simulink model "seventh"  (R2020a)
settings: Solver=VariableStepAuto  StartTime=0.0  StopTime=10.0  RelTol=1e-3
model workspace (MAT data in the model file):
  A = Simulink.Parameter
  A.Value = 1
  A.DataType = 'auto'
  A.Dimensions = [1 1]
  B = Simulink.Parameter
  B.Value = 2
  B.DataType = 'auto'
  B.Dimensions = [1 1]
  C = Simulink.Parameter
  C.Value = -1
  C.DataType = 'auto'
  C.Dimensions = [1 1]
  D = Simulink.Parameter
  D.Value = 1
  D.DataType = 'auto'
  D.Dimensions = [1 1]
  E = Simulink.Parameter
  E.Value = 1
  E.DataType = 'auto'
  E.Dimensions = [1 1]
  F = Simulink.Parameter
  F.Value = -1
  F.DataType = 'auto'
  F.Dimensions = [1 1]
settings Model: Creator=Admin  LastModifiedBy=Admin

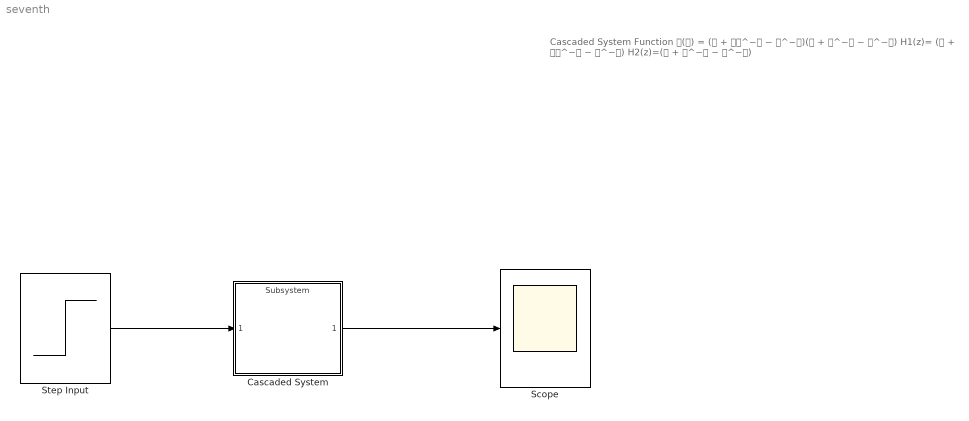
== system seventh ==
  note: Cascaded System Function
      | 𝐇(𝐳) = (𝟏 + 𝟐𝐳^−𝟏 − 𝐳^−𝟐)(𝟏 + 𝐳^−𝟏 − 𝐳^−𝟐)
      |
      | H1(z)= (𝟏 + 𝟐𝐳^−𝟏 − 𝐳^−𝟐)
      | H2(z)=(𝟏 + 𝐳^−𝟏 − 𝐳^−𝟐)
  Cascaded System : ModelReference  ModelNameDialog=Subsystem  ModelReferenceVersion=1.5
  Scope : Scope
  Step Input : Step  SampleTime=0
  wires:
  Cascaded System/1 -> Scope/1
  Step Input/1 -> Cascaded System/1
